simulink model "nid_cvst_what_is_nid_modiv"  (Simulink 8.1)
settings: Solver=FixedStepDiscrete  StartTime=0.0  StopTime=inf  RelTol=1e-3
undefined symbols (not defined in the file or in its folder): jet
libraries: visionsinks x4, nid_lib x4
settings Model: Creator=tchikama  LastModifiedBy=BeeLED
settings DataIOCC: SaveOutput=off
settings OptimizationCC: SimCompilerOptimization=On
settings HardwareCC: ProdIntDivRoundTo=Zero  ProdEndianess=LittleEndian  ProdHWDeviceType=Generic->32-bit x86 compatible
settings RTWCC: ProcessScript=grt_make_rtw_hook  RTWCompilerOptimization=On
settings CodeAppCC: MaxIdLength=95

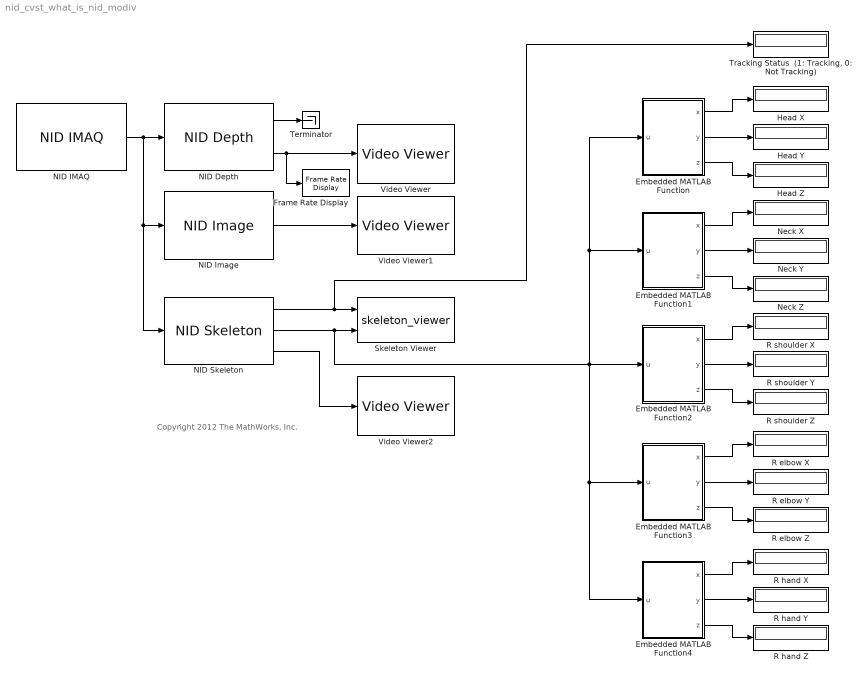
== system nid_cvst_what_is_nid_modiv ==
  note: Copyright 2012 The MathWorks, Inc.
  Embedded MATLAB Function : MATLAB Function  TreatAsAtomicUnit=on
  Embedded MATLAB Function1 : MATLAB Function  TreatAsAtomicUnit=on
  Embedded MATLAB Function2 : MATLAB Function  TreatAsAtomicUnit=on
  Embedded MATLAB Function3 : MATLAB Function  TreatAsAtomicUnit=on
  Embedded MATLAB Function4 : MATLAB Function  TreatAsAtomicUnit=on
  Frame Rate Display : visionsinks/Frame Rate Display  UpdateRate=10
  Head X : Display
  Head Y : Display
  Head Z : Display
  NID Depth : nid_lib/NID Depth  depthOutput=Depth  conv_XYZ_RW=off  viewer=on
  NID IMAQ : nid_lib/NID IMAQ  imaq_depth=on  imaq_motion=off  imaq_image=on  view_point=on  imaq_skeleton=on  imaq_ir=off  mirror_image=off  imaq_sample_time=1/30  res_fps=VGA (640x480): 30 FPS  needPsiPose=off  angle_input=off  angle=0  angle_read=off  near_mode=off  seated_mode=off  skeleton_smooth=[0.5 0.5 0.5 0.05 0.04]  infer_skeleton=on
  NID Image : nid_lib/NID Image  imageOutput=RGB
  NID Skeleton : nid_lib/NID Skeleton  num_of_skeleton_tracking=1  conv_XYZ_RW=on  viewer=on
  Neck X : Display
  Neck Y : Display
  Neck Z : Display
  R elbow X : Display
  R elbow Y : Display
  R elbow Z : Display
  R hand X : Display
  R hand Y : Display
  R hand Z : Display
  R shoulder X : Display
  R shoulder Y : Display
  R shoulder Z : Display
  Skeleton Viewer : M-S-Function  FunctionName=skeleton_viewer
      mask Display:
      | disp('Skeleton\nViewer')
      | 
      | port_label('input', 1, 'Tracking')
      | port_label('input', 2, 'Skeleton')
  Terminator : Terminator
  "Tracking Status  (1: Tracking, 0: Not Tracking)" : Display
  Video Viewer : visionsinks/Video Viewer  inputType=Obsolete7b  imagePorts=One multidimensional signal  useColorMap=off  colormapValue=jet(256)  specRange=off  minInputVal=0  maxInputVal=255  FigPos=[447 719 410 300]  AxisZoom=on  trueSizedOnce=off  OpenAtMdlStart=on  DefaultConfigurationName=vipscopes.VideoViewerScopeCfg
  Video Viewer1 : visionsinks/Video Viewer  inputType=Obsolete7b  imagePorts=One multidimensional signal  useColorMap=off  colormapValue=jet(256)  specRange=off  minInputVal=0  maxInputVal=255  FigPos=[685 615 410 300]  AxisZoom=on  trueSizedOnce=off  OpenAtMdlStart=on  DefaultConfigurationName=vipscopes.VideoViewerScopeCfg
  Video Viewer2 : visionsinks/Video Viewer  inputType=Obsolete7b  imagePorts=One multidimensional signal  useColorMap=off  colormapValue=jet(256)  specRange=off  minInputVal=0  maxInputVal=255  FigPos=[60 607 410 300]  AxisZoom=on  trueSizedOnce=off  OpenAtMdlStart=on  DefaultConfigurationName=vipscopes.VideoViewerScopeCfg
  wires:
  NID IMAQ/1 -> NID Depth/1, NID Skeleton/1, NID Image/1
  NID Skeleton/3 -> Video Viewer2/1
  NID Depth/2 -> Frame Rate Display/1, Video Viewer/1
  NID Depth/1 -> Terminator/1
  NID Image/1 -> Video Viewer1/1
  NID Skeleton/2 -> Embedded MATLAB Function3/1(u), Embedded MATLAB Function4/1(u), Embedded MATLAB Function/1(u), Embedded MATLAB Function1/1(u), Embedded MATLAB Function2/1(u), Skeleton Viewer/2
  Embedded MATLAB Function/1(x) -> Head X/1
  Embedded MATLAB Function/2(y) -> Head Y/1
  Embedded MATLAB Function/3(z) -> Head Z/1
  Embedded MATLAB Function1/1(x) -> Neck X/1
  Embedded MATLAB Function1/2(y) -> Neck Y/1
  Embedded MATLAB Function1/3(z) -> Neck Z/1
  Embedded MATLAB Function2/1(x) -> R shoulder X/1
  Embedded MATLAB Function2/2(y) -> R shoulder Y/1
  Embedded MATLAB Function2/3(z) -> R shoulder Z/1
  Embedded MATLAB Function3/1(x) -> R elbow X/1
  Embedded MATLAB Function3/2(y) -> R elbow Y/1
  Embedded MATLAB Function3/3(z) -> R elbow Z/1
  Embedded MATLAB Function4/1(x) -> R hand X/1
  Embedded MATLAB Function4/2(y) -> R hand Y/1
  Embedded MATLAB Function4/3(z) -> R hand Z/1
  NID Skeleton/1 -> "Tracking Status  (1: Tracking, 0: Not Tracking)"/1, Skeleton Viewer/1

== matlab function Embedded MATLAB Function1 ==
  data: x output double; u input double; y output double; z output double
function [x,y,z] = fcn(u)
%#eml

%
% Neck
%
if length(u) == 20
    idx = 3; % Kinect SDK
else
    idx = 2; % OpenNI
end

x = u(:,idx,1);
y = u(:,idx,2);
z = u(:,idx,3);

== matlab function Embedded MATLAB Function ==
  data: x output double; u input double; y output double; z output double
function [x,y,z] = fcn(u)
%#eml

%
% Head
%
if length(u) == 20
    idx = 4; % Kinect SDK
else
    idx = 1; % OpenNI
end

x = u(:,idx,1);
y = u(:,idx,2);
z = u(:,idx,3);

== matlab function Embedded MATLAB Function2 ==
  data: x output double; u input double; y output double; z output double
function [x,y,z] = fcn(u)
%#eml

%
% Right shoulder
%
if length(u) == 20
    idx = 9; % Kinect SDK
else
    idx = 4; % OpenNI
end

x = u(:,idx,1);
y = u(:,idx,2);
z = u(:,idx,3);

== matlab function Embedded MATLAB Function3 ==
  data: x output double; u input double; y output double; z output double
function [x,y,z] = fcn(u)
%#eml

%
% Right elbow
%
if length(u) == 20
    idx = 10; % Kinect SDK
else
    idx = 5; % OpenNI
end

x = u(:,idx,1);
y = u(:,idx,2);
z = u(:,idx,3);

== matlab function Embedded MATLAB Function4 ==
  data: x output double; u input double; y output double; z output double
function [x,y,z] = fcn(u)
%#eml

%
% Right hand
%
if length(u) == 20
    idx = 12; % Kinect SDK
else
    idx = 6; % OpenNI
end

x = u(:,idx,1);
y = u(:,idx,2);
z = u(:,idx,3);
